simulink model "lt_sim"  (R2020a)
settings: Solver=VariableStepAuto  StartTime=0.0  StopTime=10  RelTol=1e-3
libraries: fl_lib x28, nesl_utility x5, simulink x1, ee_lib x1
settings Model: Creator=sujit  LastModifiedBy=sujit

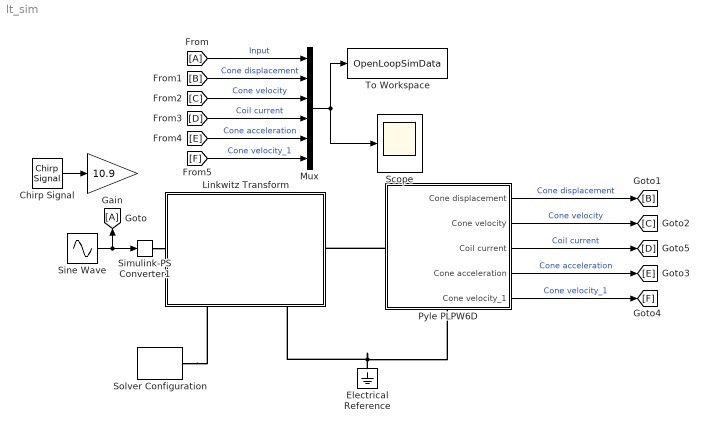
== system lt_sim ==
  Chirp Signal : simulink/Sources/Chirp Signal  f1=20  T=10  f2=1000
  Electrical Reference : fl_lib/Electrical/Electrical Elements/Electrical Reference
      settings: SourceProductBaseCode=MT,SS
  Gain : Gain  Gain=10.9
  Linkwitz Transform : Subsystem
      settings: PortSchema="{\"entries\":[{\"content\":{\"sides\":[{\"content\":{\"connectorIds\":[\"LConn1\"]},\"type\":\"ConnectorPlacement.EquallySpacedRectSide\",\"uuid\":\"c176afcd-22cf-4a96-95a5-2f4a01c27625\"},{\"content\":{\"connectorIds\":[\"RConn1\"],\"side\":\"RIGHT\"},\"type\":\"ConnectorPlacement.EquallySpacedRectSide\",\"uuid\":\"3d91d6b3-2fcd-4fa9-a9e2-01e15fe19188\"},{\"content\":{\"connectorIds\":[],\"side\":\"TOP\"},\"type\":\"ConnectorPlacement.EquallySpacedRectSide\",\"uuid\":\"62fa6f1b-807a-445e-accc-cb6b6c056347\"},{\"content\":{\"connectorIds\":[\"RConn2\",\"RConn3\"],\"side\":\"BOTTOM\"},\"type\":\"ConnectorPlacement.EquallySpacedRectSide\",\"uuid\":\"aba00412-b7f6-420c-bbf2-ad0cfa3564f9\"}]},\"type\":\"ConnectorPlacement.EquallySpacedConnector\",\"uuid\":\"560b3fee-5e65-4d46-bef7-272889515bf8\"}],\"packageUris\":[\"http://schema.mathworks.com/mf0/Connector/19700101\"],\"version\":\"1.0\"}"
      mask Display: image('/Users/sujit/Documents/UNIVERSITY/3rd Year Project/git/3rd-year-project/Images/LT.png'); % Use "Edit Image" on toolstrip to change.
  Mux : Mux  Inputs=6
  Pyle PLPW6D : Subsystem
      settings: PortSchema="{\"entries\":[{\"content\":{\"sides\":[{\"content\":{\"connectorIds\":[\"LConn1\"]},\"type\":\"ConnectorPlacement.EquallySpacedRectSide\",\"uuid\":\"55797129-f68c-4c08-9179-5bd73ddaf456\"},{\"content\":{\"connectorIds\":[\"Out1\",\"Out2\",\"Out3\",\"Out4\",\"Out5\"],\"side\":\"RIGHT\"},\"type\":\"ConnectorPlacement.EquallySpacedRectSide\",\"uuid\":\"cd82eb0c-b61b-42dc-852e-e59ea1718ce1\"},{\"content\":{\"connectorIds\":[],\"side\":\"TOP\"},\"type\":\"ConnectorPlacement.EquallySpacedRectSide\",\"uuid\":\"8a8988be-8c05-45b5-a601-761f58a02f2f\"},{\"content\":{\"connectorIds\":[\"RConn1\"],\"side\":\"BOTTOM\"},\"type\":\"ConnectorPlacement.EquallySpacedRectSide\",\"uuid\":\"149d6272-c2cd-47e3-ba3f-f898f69521a5\"}]},\"type\":\"ConnectorPlacement.EquallySpacedConnector\",\"uuid\":\"fa7a078c-6bab-4c84-8cb9-27fcf7a24b1b\"}],\"packageUris\":[\"http://schema.mathworks.com/mf0/Connector/19700101\"],\"version\":\"1.0\"}"
      mask Display: image('/Users/sujit/Documents/UNIVERSITY/3rd Year Project/git/3rd-year-project/Images/PLPW6D.jpg'); % Use "Edit Image" on toolstrip to change.
  Scope : Scope
  Simulink-PS Converter1 : nesl_utility/Simulink-PS Converter  PhysicalDomain=network_engine_domain  SubClassName=ps_input  LeftPortType=input  RightPortType=output  PseudoPeriodic=off  Frequencies=[]  NoiseDistribution=none  NoiseParameters=[]  Unit=1  AffineConversion=off  FilteringAndDerivatives=provide  SimscapeFilterOrder=1  InputFilterTimeConstant=0.001  UdotUserProvided=0
  Sine Wave : Sin  Amplitude=10.9  Frequency=125  SampleTime=0
  Solver Configuration : nesl_utility/Solver Configuration  PhysicalDomain=network_engine_domain  SubClassName=solver  LeftPortType=input  RightPortType=generic  Tones=[]  Harmonics=[]  SimulateNoise=off  Profile=off  UseLocalSampling=off  EnableSwitchedLinearOptims=on  FrequencyDomain=off  UseCCode=off  RelTol=0.001  AbsTol=1e-06  MinStep=1e-09  ToWorkspace=off  RevertToSquareIcSolve=off  NumHomotopyIterations=100  PhasorMode=off  PhasorModeNumHarmonics=1  DoDC=off  ResidualTolerance=1e-09  UseLocalSolver=off  LocalSolverChoice=NE_BACKWARD_EULER_ADVANCER  LocalSolverSampleTime=0.001  DoFixedCost=off  MaxNonlinIter=3  MaxModeIter=2  LinearAlgebra=auto  EquationFormulation=NE_TIME_EF  DelaysMemoryBudget=1024  AutomaticFiltering=on  FilteringTimeConstant=0.001  PartitionStorageMethod=AS_NEEDED  PartitionMemoryBudget=1024  PartitionMethod=ROBUST
  To Workspace : ToWorkspace  VariableName=OpenLoopSimData  SaveFormat=Timeseries  SampleTime=-1
  wires:
  Chirp Signal/1 -> Gain/1
  [A] -> Mux/1  "Input"
  [B] -> Mux/2  "Cone displacement"
  [C] -> Mux/3  "Cone velocity"
  [D] -> Mux/4  "Coil current"
  Mux/1 -> Scope/1, To Workspace/1
  [E] -> Mux/5  "Cone acceleration"
  Sine Wave/1 -> Simulink-PS Converter1/1, [A]
  Pyle PLPW6D/3(Coil current) -> [D]  "Coil current"
  Pyle PLPW6D/1(Cone displacement) -> [B]  "Cone displacement"
  Pyle PLPW6D/2(Cone velocity) -> [C]  "Cone velocity"
  Pyle PLPW6D/4(Cone acceleration) -> [E]  "Cone acceleration"
  Pyle PLPW6D/5(Cone velocity_1) -> [F]  "Cone velocity_1"
  [F] -> Mux/6  "Cone velocity_1"
  connections:
  Simulink-PS Converter1/RConn1 -- Linkwitz Transform/LConn1
  Solver Configuration/RConn1 -- Linkwitz Transform/RConn2
  Electrical Reference/LConn1 -- Linkwitz Transform/RConn3 -- Pyle PLPW6D/RConn1
  Pyle PLPW6D/LConn1 -- Linkwitz Transform/RConn1

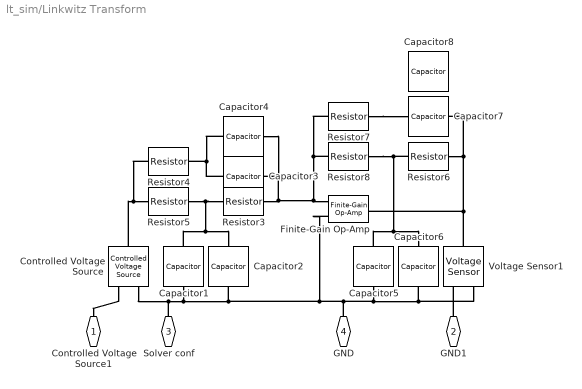
== system lt_sim/Linkwitz Transform ==
  Capacitor1 : fl_lib/Electrical/Electrical Elements/Capacitor  c=150 nF  r=0 Ohm  g=0 1/Ohm  i_specify=off  i_priority=None  i=0 A  i_nominal_specify=off  i_nominal_unit=A  i_nominal_value=1  v_specify=off  v_priority=None  v=0 V  v_nominal_specify=off  v_nominal_unit=V  v_nominal_value=1  vc_specify=off  vc_priority=High  vc=0 V  vc_nominal_specify=off  vc_nominal_unit=V  vc_nominal_value=1
  Capacitor2 : fl_lib/Electrical/Electrical Elements/Capacitor  c=47 nF  r=0 Ohm  g=0 1/Ohm  i_specify=off  i_priority=None  i=0 A  i_nominal_specify=off  i_nominal_unit=A  i_nominal_value=1  v_specify=off  v_priority=None  v=0 V  v_nominal_specify=off  v_nominal_unit=V  v_nominal_value=1  vc_specify=off  vc_priority=High  vc=0 V  vc_nominal_specify=off  vc_nominal_unit=V  vc_nominal_value=1
  Capacitor3 : fl_lib/Electrical/Electrical Elements/Capacitor  c=22 nF  r=0 Ohm  g=0 1/Ohm  i_specify=off  i_priority=None  i=0 A  i_nominal_specify=off  i_nominal_unit=A  i_nominal_value=1  v_specify=off  v_priority=None  v=0 V  v_nominal_specify=off  v_nominal_unit=V  v_nominal_value=1  vc_specify=off  vc_priority=High  vc=0 V  vc_nominal_specify=off  vc_nominal_unit=V  vc_nominal_value=1
  Capacitor4 : fl_lib/Electrical/Electrical Elements/Capacitor  c=47 nF  r=0 Ohm  g=0 1/Ohm  i_specify=off  i_priority=None  i=0 A  i_nominal_specify=off  i_nominal_unit=A  i_nominal_value=1  v_specify=off  v_priority=None  v=0 V  v_nominal_specify=off  v_nominal_unit=V  v_nominal_value=1  vc_specify=off  vc_priority=High  vc=0 V  vc_nominal_specify=off  vc_nominal_unit=V  vc_nominal_value=1
  Capacitor5 : fl_lib/Electrical/Electrical Elements/Capacitor  c=6.8 nF  r=0 Ohm  g=0 1/Ohm  i_specify=off  i_priority=None  i=0 A  i_nominal_specify=off  i_nominal_unit=A  i_nominal_value=1  v_specify=off  v_priority=None  v=0 V  v_nominal_specify=off  v_nominal_unit=V  v_nominal_value=1  vc_specify=off  vc_priority=High  vc=0 V  vc_nominal_specify=off  vc_nominal_unit=V  vc_nominal_value=1
  Capacitor6 : fl_lib/Electrical/Electrical Elements/Capacitor  c=470 pF  r=0 Ohm  g=0 1/Ohm  i_specify=off  i_priority=None  i=0 A  i_nominal_specify=off  i_nominal_unit=A  i_nominal_value=1  v_specify=off  v_priority=None  v=0 V  v_nominal_specify=off  v_nominal_unit=V  v_nominal_value=1  vc_specify=off  vc_priority=High  vc=0 V  vc_nominal_specify=off  vc_nominal_unit=V  vc_nominal_value=1
  Capacitor7 : fl_lib/Electrical/Electrical Elements/Capacitor  c=62 nF  r=0 Ohm  g=0 1/Ohm  i_specify=off  i_priority=None  i=0 A  i_nominal_specify=off  i_nominal_unit=A  i_nominal_value=1  v_specify=off  v_priority=None  v=0 V  v_nominal_specify=off  v_nominal_unit=V  v_nominal_value=1  vc_specify=off  vc_priority=High  vc=0 V  vc_nominal_specify=off  vc_nominal_unit=V  vc_nominal_value=1
  Capacitor8 : fl_lib/Electrical/Electrical Elements/Capacitor  c=47 nF  r=0 Ohm  g=0 1/Ohm  i_specify=off  i_priority=None  i=0 A  i_nominal_specify=off  i_nominal_unit=A  i_nominal_value=1  v_specify=off  v_priority=None  v=0 V  v_nominal_specify=off  v_nominal_unit=V  v_nominal_value=1  vc_specify=off  vc_priority=High  vc=0 V  vc_nominal_specify=off  vc_nominal_unit=V  vc_nominal_value=1
  Controlled Voltage Source : fl_lib/Electrical/Electrical Sources/Controlled Voltage Source
  Finite-Gain Op-Amp : ee_lib/Integrated Circuits/Finite-Gain Op-Amp  A=1000  Rin=1e12 Ohm  Rout=100 Ohm  Vmin=-12 V  Vmax=12 V  noise_mode=0  v_noise=30e-9 V/Hz^0.50000  noise_prm=1  i_noise=0.5e-12 A/Hz^0.50000  ip_noise=0.5e-12 A/Hz^0.50000  in_noise=0.5e-12 A/Hz^0.50000  sample_time=1e-3 s  repeatability=1  auto_seed_v=2812350261  auto_seed_ip=2528642791  auto_seed_in=3199986473  user_seed_v=0  user_seed_ip=0  user_seed_in=0
      settings: SourceProductBaseCode=PS  InternalSimscapePortConfiguration="{\"Bottom\":[],\"Left\":[{\"id\":\"p\",\"label\":\"+\",\"type\":\"foundation.electrical.electrical\"},{\"id\":\"n\",\"label\":\"-\",\"type\":\"foundation.electrical.electrical\"}],\"Right\":[{\"id\":\"out\",\"label\":\"\",\"type\":\"foundation.electrical.electrical\"}],\"Top\":[]}"
  Resistor3 : fl_lib/Electrical/Electrical Elements/Resistor  R=15.4 kOhm  i_specify=off  i_priority=None  i=0 A  i_nominal_specify=off  i_nominal_unit=A  i_nominal_value=1  v_specify=off  v_priority=None  v=0 V  v_nominal_specify=off  v_nominal_unit=V  v_nominal_value=1
  Resistor4 : fl_lib/Electrical/Electrical Elements/Resistor  R=13.3 kOhm  i_specify=off  i_priority=None  i=0 A  i_nominal_specify=off  i_nominal_unit=A  i_nominal_value=1  v_specify=off  v_priority=None  v=0 V  v_nominal_specify=off  v_nominal_unit=V  v_nominal_value=1
  Resistor5 : fl_lib/Electrical/Electrical Elements/Resistor  R=15.4 kOhm  i_specify=off  i_priority=None  i=0 A  i_nominal_specify=off  i_nominal_unit=A  i_nominal_value=1  v_specify=off  v_priority=None  v=0 V  v_nominal_specify=off  v_nominal_unit=V  v_nominal_value=1
  Resistor6 : fl_lib/Electrical/Electrical Elements/Resistor  R=442 kOhm  i_specify=off  i_priority=None  i=0 A  i_nominal_specify=off  i_nominal_unit=A  i_nominal_value=1  v_specify=off  v_priority=None  v=0 V  v_nominal_specify=off  v_nominal_unit=V  v_nominal_value=1
  Resistor7 : fl_lib/Electrical/Electrical Elements/Resistor  R=13.3 kOhm  i_specify=off  i_priority=None  i=0 A  i_nominal_specify=off  i_nominal_unit=A  i_nominal_value=1  v_specify=off  v_priority=None  v=0 V  v_nominal_specify=off  v_nominal_unit=V  v_nominal_value=1
  Resistor8 : fl_lib/Electrical/Electrical Elements/Resistor  R=442 kOhm  i_specify=off  i_priority=None  i=0 A  i_nominal_specify=off  i_nominal_unit=A  i_nominal_value=1  v_specify=off  v_priority=None  v=0 V  v_nominal_specify=off  v_nominal_unit=V  v_nominal_value=1
  Voltage Sensor1 : fl_lib/Electrical/Electrical Sensors/Voltage Sensor
  Controlled Voltage Source1 : PMIOPort  Side=Left
  GND1 : PMIOPort  Port=2  Side=Right
  Solver conf : PMIOPort  Port=3  Side=Right
  GND : PMIOPort  Port=4  Side=Right
  connections:
  Resistor7/RConn1 -- Capacitor7/LConn1
  Resistor3/LConn1 -- Resistor5/RConn1 -- Capacitor1/LConn1 -- Capacitor2/LConn1
  Capacitor3/LConn1 -- Capacitor4/LConn1 -- Resistor4/RConn1
  Resistor8/RConn1 -- Resistor6/LConn1 -- Capacitor5/LConn1 -- Capacitor6/LConn1
  Capacitor5/RConn1 -- Solver conf/RConn1 -- Controlled Voltage Source/RConn2 -- Capacitor1/RConn1 -- Capacitor2/RConn1 -- Finite-Gain Op-Amp/LConn1 -- GND/RConn1 -- Voltage Sensor1/RConn2 -- Capacitor6/RConn1
  Resistor3/RConn1 -- Finite-Gain Op-Amp/LConn2 -- Resistor7/LConn1 -- Resistor8/LConn1 -- Capacitor4/RConn1 -- Capacitor3/RConn1
  Controlled Voltage Source/RConn1 -- Controlled Voltage Source1/RConn1
  Capacitor7/RConn1 -- Voltage Sensor1/LConn1 -- Finite-Gain Op-Amp/RConn1 -- Resistor6/RConn1
  Resistor4/LConn1 -- Controlled Voltage Source/LConn1 -- Resistor5/LConn1
  GND1/RConn1 -- Voltage Sensor1/RConn1

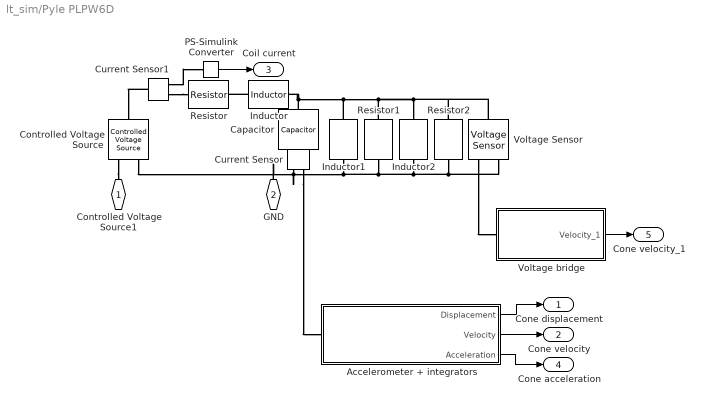
== system lt_sim/Pyle PLPW6D ==
  Accelerometer + integrators : Subsystem
  Capacitor : fl_lib/Electrical/Electrical Elements/Capacitor  c=388.95 uF  r=0 Ohm  g=0 1/Ohm  i_specify=off  i_priority=None  i=0 A  i_nominal_specify=off  i_nominal_unit=A  i_nominal_value=1  v_specify=off  v_priority=None  v=0 V  v_nominal_specify=off  v_nominal_unit=V  v_nominal_value=1  vc_specify=off  vc_priority=High  vc=0 V  vc_nominal_specify=off  vc_nominal_unit=V  vc_nominal_value=1
  Controlled Voltage Source : fl_lib/Electrical/Electrical Sources/Controlled Voltage Source
  Current Sensor : fl_lib/Electrical/Electrical Sensors/Current Sensor
  Current Sensor1 : fl_lib/Electrical/Electrical Sensors/Current Sensor
  Inductor : fl_lib/Electrical/Electrical Elements/Inductor  l=148.8 uH  r=0 Ohm  g=0 1/Ohm  i_specify=off  i_priority=None  i=0 A  i_nominal_specify=off  i_nominal_unit=A  i_nominal_value=1  v_specify=off  v_priority=None  v=0 V  v_nominal_specify=off  v_nominal_unit=V  v_nominal_value=1  i_L_specify=off  i_L_priority=High  i_L=0 A  i_L_nominal_specify=off  i_L_nominal_unit=A  i_L_nominal_value=1
  Inductor1 : fl_lib/Electrical/Electrical Elements/Inductor  l=23.9 mH  r=0 Ohm  g=0 1/Ohm  i_specify=off  i_priority=None  i=0 A  i_nominal_specify=off  i_nominal_unit=A  i_nominal_value=1  v_specify=off  v_priority=None  v=0 V  v_nominal_specify=off  v_nominal_unit=V  v_nominal_value=1  i_L_specify=off  i_L_priority=High  i_L=0 A  i_L_nominal_specify=off  i_L_nominal_unit=A  i_L_nominal_value=1
  Inductor2 : fl_lib/Electrical/Electrical Elements/Inductor  l=9 mH  r=0 Ohm  g=0 1/Ohm  i_specify=off  i_priority=None  i=0 A  i_nominal_specify=off  i_nominal_unit=A  i_nominal_value=1  v_specify=off  v_priority=None  v=0 V  v_nominal_specify=off  v_nominal_unit=V  v_nominal_value=1  i_L_specify=off  i_L_priority=High  i_L=0 A  i_L_nominal_specify=off  i_L_nominal_unit=A  i_L_nominal_value=1
  PS-Simulink Converter : nesl_utility/PS-Simulink Converter  PhysicalDomain=network_engine_domain  SubClassName=ps_output  LeftPortType=input  RightPortType=output  PseudoPeriodic=off  Frequencies=[]  Unit=inherit  AffineConversion=off
  Resistor : fl_lib/Electrical/Electrical Elements/Resistor  R=3.4 Ohm  i_specify=off  i_priority=None  i=0 A  i_nominal_specify=off  i_nominal_unit=A  i_nominal_value=1  v_specify=off  v_priority=None  v=0 V  v_nominal_specify=off  v_nominal_unit=V  v_nominal_value=1
  Resistor1 : fl_lib/Electrical/Electrical Elements/Resistor  R=28.42 Ohm  i_specify=off  i_priority=None  i=0 A  i_nominal_specify=off  i_nominal_unit=A  i_nominal_value=1  v_specify=off  v_priority=None  v=0 V  v_nominal_specify=off  v_nominal_unit=V  v_nominal_value=1
  Resistor2 : fl_lib/Electrical/Electrical Elements/Resistor  R=282 Ohm  i_specify=off  i_priority=None  i=0 A  i_nominal_specify=off  i_nominal_unit=A  i_nominal_value=1  v_specify=off  v_priority=None  v=0 V  v_nominal_specify=off  v_nominal_unit=V  v_nominal_value=1
  Voltage Sensor : fl_lib/Electrical/Electrical Sensors/Voltage Sensor
  Voltage bridge : Subsystem
  Controlled Voltage Source1 : PMIOPort  Side=Left
  GND : PMIOPort  Port=2  Side=Right
  Cone displacement : Outport
  Cone velocity : Outport  Port=2
  Coil current : Outport  Port=3
  Cone acceleration : Outport  Port=4
  Cone velocity_1 : Outport  Port=5
  wires:
  Accelerometer + integrators/1(Displacement) -> Cone displacement/1
  Accelerometer + integrators/2(Velocity) -> Cone velocity/1
  PS-Simulink Converter/1 -> Coil current/1
  Accelerometer + integrators/3(Acceleration) -> Cone acceleration/1
  Voltage bridge/1(Velocity_1) -> Cone velocity_1/1
  connections:
  Voltage Sensor/RConn1 -- Voltage bridge/LConn1
  Controlled Voltage Source/RConn1 -- Controlled Voltage Source1/RConn1
  Resistor2/RConn1 -- Voltage Sensor/RConn2 -- Inductor2/RConn1 -- Resistor1/RConn1 -- Current Sensor/RConn2 -- Controlled Voltage Source/RConn2 -- GND/RConn1 -- Inductor1/RConn1
  Capacitor/RConn1 -- Current Sensor/LConn1
  Current Sensor/RConn1 -- Accelerometer + integrators/LConn1
  Capacitor/LConn1 -- Inductor1/LConn1 -- Inductor2/LConn1 -- Voltage Sensor/LConn1 -- Resistor2/LConn1 -- Resistor1/LConn1 -- Inductor/RConn1
  Inductor/LConn1 -- Resistor/RConn1
  Current Sensor1/RConn2 -- Resistor/LConn1
  Current Sensor1/LConn1 -- Controlled Voltage Source/LConn1
  Current Sensor1/RConn1 -- PS-Simulink Converter/LConn1

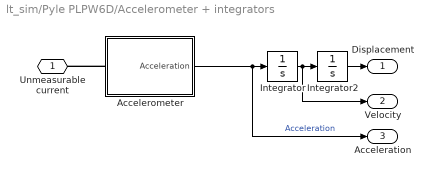
== system lt_sim/Pyle PLPW6D/Accelerometer + integrators ==
  Accelerometer : Subsystem
  Integrator : Integrator
  Integrator2 : Integrator
  Unmeasurable current : PMIOPort  Side=Left
  Displacement : Outport
  Velocity : Outport  Port=2
  Acceleration : Outport  Port=3
  wires:
  Integrator2/1 -> Displacement/1
  Integrator/1 -> Velocity/1, Integrator2/1
  Accelerometer/1(Acceleration) -> Acceleration/1, Integrator/1  "Acceleration"
  connections:
  Accelerometer/LConn1 -- Unmeasurable current/RConn1

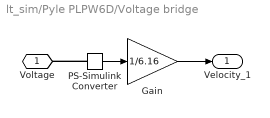
== system lt_sim/Pyle PLPW6D/Voltage bridge ==
  Gain : Gain  Gain=1/6.16
  PS-Simulink Converter : nesl_utility/PS-Simulink Converter  PhysicalDomain=network_engine_domain  SubClassName=ps_output  LeftPortType=input  RightPortType=output  PseudoPeriodic=off  Frequencies=[]  Unit=inherit  AffineConversion=off
  Voltage : PMIOPort  Side=Left
  Velocity_1 : Outport
  wires:
  PS-Simulink Converter/1 -> Gain/1
  Gain/1 -> Velocity_1/1
  connections:
  PS-Simulink Converter/LConn1 -- Voltage/RConn1

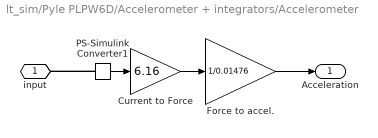
== system lt_sim/Pyle PLPW6D/Accelerometer + integrators/Accelerometer ==
  Current to Force : Gain  Gain=6.16
  Force to accel. : Gain  Gain=1/0.01476
  PS-Simulink Converter1 : nesl_utility/PS-Simulink Converter  PhysicalDomain=network_engine_domain  SubClassName=ps_output  LeftPortType=input  RightPortType=output  PseudoPeriodic=off  Frequencies=[]  Unit=inherit  AffineConversion=off
  input : PMIOPort  Side=Left
  Acceleration : Outport
  wires:
  Force to accel./1 -> Acceleration/1
  Current to Force/1 -> Force to accel./1
  PS-Simulink Converter1/1 -> Current to Force/1
  connections:
  PS-Simulink Converter1/LConn1 -- input/RConn1
